simulink model "Module_8"  (R2018a)
settings: Solver=VariableStepAuto  StartTime=0.0  StopTime=10.0  RelTol=1e-3
undefined symbols (not defined in the file): Cg, Cs, k, kc, kg, kr, simSwitch, u0, v0, x0
settings Model: Creator=pala  LastModifiedBy=pala
settings DataIOCC: SaveFinalState=on  SaveFormat=StructureWithTime  SaveState=on

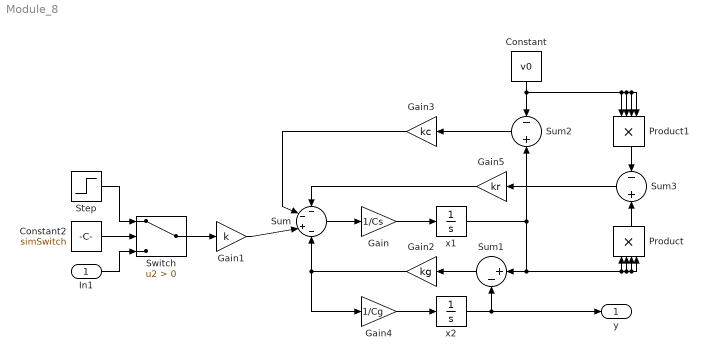
== system Module_8 ==
  In1 : Inport
  Constant : Constant  Value=v0
  Constant2 : Constant  Value=simSwitch
  Gain : Gain  Gain=1/Cs
  Gain1 : Gain  Gain=k
  Gain2 : Gain  Gain=kg
  Gain3 : Gain  Gain=kc
  Gain4 : Gain  Gain=1/Cg
  Gain5 : Gain  Gain=kr
  Product : Product  Inputs=4
  Product1 : Product  Inputs=4
  Step : Step  After=u0  SampleTime=0
  Sum : Sum  Inputs=--+-
  Sum1 : Sum  Inputs=|+-
  Sum2 : Sum  Inputs=-|+
  Sum3 : Sum  Inputs=-|+
  Switch : Switch  Criteria=u2 > Threshold
  x1 : Integrator  Priority=1  InitialCondition=x0(1)
  x2 : Integrator  Priority=2  InitialCondition=x0(2)
  y : Outport
  wires:
  Gain/1 -> x1/1
  Sum/1 -> Gain/1
  x1/1 -> Sum2/2, Sum1/1, Product/1, Product/2, Product/3, Product/4
  x2/1 -> y/1, Sum1/2
  Sum1/1 -> Gain2/1
  Gain1/1 -> Sum/3
  Gain2/1 -> Gain4/1, Sum/4
  Constant/1 -> Product1/1, Product1/2, Product1/3, Product1/4, Sum2/1
  Sum2/1 -> Gain3/1
  Gain3/1 -> Sum/2
  Sum3/1 -> Gain5/1
  Gain4/1 -> x2/1
  Gain5/1 -> Sum/1
  Constant2/1 -> Switch/2
  Step/1 -> Switch/1
  In1/1 -> Switch/3
  Switch/1 -> Gain1/1
  Product1/1 -> Sum3/1
  Product/1 -> Sum3/2
